simulink model "mod_05"  (R2017b)
settings: Solver=VariableStepAuto  StartTime=0.0  StopTime=10.0  RelTol=1e-3
values from neighbouring files (symbols this model uses):
  a = -(c*d)/b    [file_05.m]    (also in file_05_04.m)
  b = (c+d)/2    [file_05.m]    (also in file_05_04.m)
  c = -1+3i    [file_05.m]    (also in file_05_04.m = -1+i)
  d = -1-3i    [file_05.m]    (also in file_05_04.m = -1-i)
settings Model: Creator=Manu  LastModifiedBy=Manu

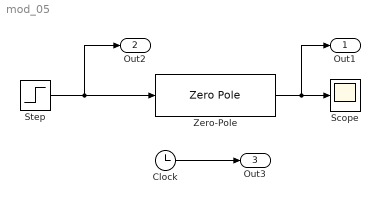
== system mod_05 ==
  Clock : Clock
  Scope : Scope
  Step : Step  SampleTime=0
  Zero-Pole : ZeroPole  Zeros=[b]  Poles=[0 c d]  Gain=[a]
  Out1 : Outport
  Out2 : Outport  Port=2
  Out3 : Outport  Port=3
  wires:
  Clock/1 -> Out3/1
  Step/1 -> Zero-Pole/1, Out2/1
  Zero-Pole/1 -> Out1/1, Scope/1
